simulink model "juros"  (R2024b)
settings: Solver=VariableStepAuto  StartTime=0.0  StopTime=10.0  RelTol=1e-3
settings Model: Creator=jackn  LastModifiedBy=jackn

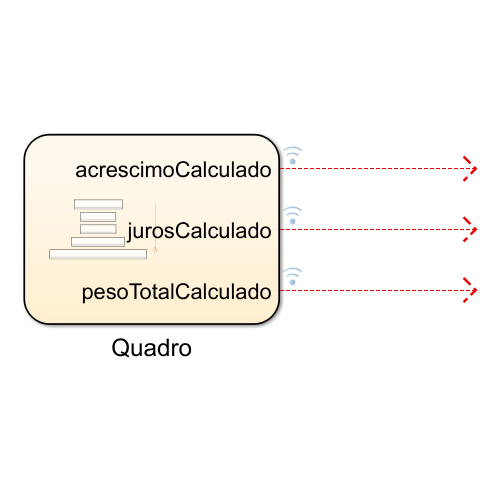
[thumbnail: Simulink's stored preview of the top-level diagram]
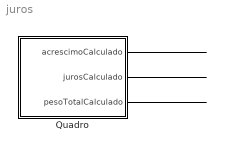
== system juros ==
  Quadro : Stateflow chart  TreatAsAtomicUnit=on
  wires:
  Quadro/1(acrescimoCalculado) -> ?
  Quadro/2(jurosCalculado) -> ?
  Quadro/3(pesoTotalCalculado) -> ?

== matlab function juros/Quadro ==
  data: indice function_input; pagamento function_output; unused function_input; peso function_output; pesoTotal function_output; juros function_input; acrescimo function_output; acrescimo function_input; precisao function_input; maxIteracoes function_input; maxJuros function_input; juros function_output; Composto constant boolean =true; Periodo constant double =30.0; Quantidade constant int32 =3; acrescimoCalculado output; jurosCalculado output; pesoTotalCalculado output
function pagamento = Pagamentos(indice)
    pagamento = double(indice) * 30.0;

== matlab function juros/Quadro ==
function peso = Pesos(~)
    peso = 1.0;

== matlab function juros/Quadro ==
function pesoTotal = getPesoTotal
    acumulador = 0.0;
    for indice = 1 : Quantidade
        acumulador = acumulador + Pesos(indice);
    end
    pesoTotal = acumulador;

== matlab function juros/Quadro ==
function acrescimo = jurosParaAcrescimo(juros)
    pesoTotal = getPesoTotal();
    if juros <= 0.0 | Quantidade <= 0 | Periodo <= 0.0 | pesoTotal <= 0.0
        acrescimo = 0.0;
        return;
        end
    acumulador = 0.0;

    for indice = 1 : Quantidade
        if Composto
            acumulador = acumulador + Pesos(indice) / (1.0 + juros / 100.0) ^ (Pagamentos(indice) / Periodo);
        else
            acumulador = acumulador + Pesos(indice) / (1.0 + juros / 100.0 * Pagamentos(indice) / Periodo);
        end
    end

    if acumulador <= 0.0
        acrescimo = 0.0;
        return;
    end
    acrescimo = (pesoTotal / acumulador - 1) * 100;

== matlab function juros/Quadro ==
function juros = acrescimoParaJuros(acrescimo, precisao, maxIteracoes, maxJuros)
    pesoTotal = getPesoTotal;
    if maxIteracoes < 1 | Quantidade < 1 | precisao < 1 | Periodo <= 0.0 | acrescimo <= 0.0 | maxJuros <= 0.0 | pesoTotal <= 0.0
        juros = 0.0;
        return;
    end

    minJuros = 0.0;
    medJuros = maxJuros / 2;
    minDiferenca = 0.1 ^ precisao;
    for indice = 1 : maxIteracoes
        medJuros = (minJuros + maxJuros) / 2;
        if (maxJuros - minJuros) < minDiferenca
            juros = medJuros;
            return;
        end
        if jurosParaAcrescimo(medJuros) < acrescimo
            minJuros = medJuros;
        else
            maxJuros = medJuros;
        end
    end

    juros = medJuros;
